simulink model "Lead_Lag"  (R2022a)
settings: Solver=VariableStepAuto  StartTime=0.0  StopTime=100  RelTol=1e-3
settings Model: Creator=Alireza  LastModifiedBy=Alireza

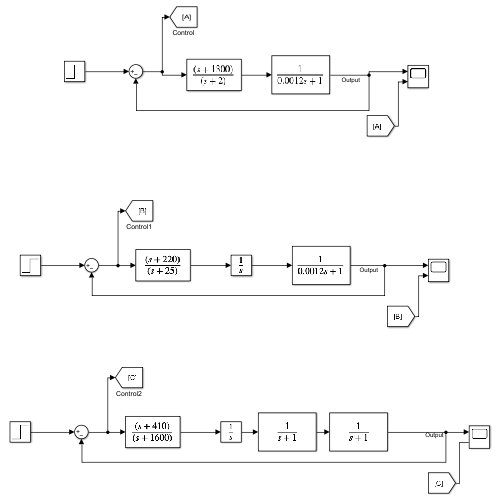
[thumbnail: Simulink's stored preview of the top-level diagram]
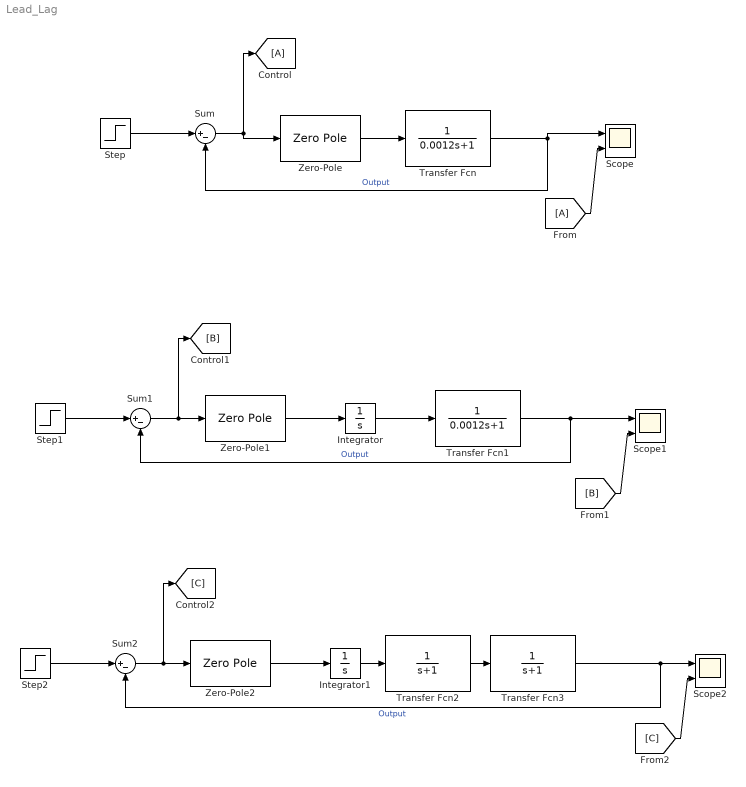
== system Lead_Lag ==
  Control : Goto
  From : From
  Integrator : Integrator
  Integrator1 : Integrator
  Scope : Scope  NumInputPorts=2
  Scope1 : Scope  NumInputPorts=2
  Scope2 : Scope  NumInputPorts=2
  Step : Step  Time=0  SampleTime=0
  Step1 : Step  Time=0  SampleTime=0
  Step2 : Step  Time=0  SampleTime=0
  Sum : Sum  Inputs=|+-
  Sum1 : Sum  Inputs=|+-
  Sum2 : Sum  Inputs=|+-
  Transfer Fcn : TransferFcn  Denominator=[0.0012 1]
  Transfer Fcn1 : TransferFcn  Denominator=[0.0012 1]
  Transfer Fcn2 : TransferFcn  Denominator=[1 1]
  Transfer Fcn3 : TransferFcn  Denominator=[1 1]
  Zero-Pole : ZeroPole  Zeros=[-1300]  Poles=[-2]
  Zero-Pole1 : ZeroPole  Zeros=[-220]  Poles=[-25]
  Zero-Pole2 : ZeroPole  Zeros=[-410]  Poles=[-1600]
  wires:
  Transfer Fcn/1 -> Sum/2, Scope/1  "Output"
  Step/1 -> Sum/1
  Sum/1 -> Control/1, Zero-Pole/1
  Zero-Pole/1 -> Transfer Fcn/1
  From/1 -> Scope/2
  Transfer Fcn1/1 -> Scope1/1, Sum1/2  "Output"
  [B] -> Scope1/2
  Step1/1 -> Sum1/1
  Sum1/1 -> Zero-Pole1/1, [B]
  Integrator/1 -> Transfer Fcn1/1
  Zero-Pole1/1 -> Integrator/1
  Step2/1 -> Sum2/1
  Transfer Fcn2/1 -> Transfer Fcn3/1
  Integrator1/1 -> Transfer Fcn2/1
  Sum2/1 -> Zero-Pole2/1, [C]
  [C] -> Scope2/2
  Transfer Fcn3/1 -> Scope2/1, Sum2/2  "Output"
  Zero-Pole2/1 -> Integrator1/1
